simulink model "brake_acc_nodiv"  (Simulink 8.6)
settings: Solver=FixedStepDiscrete  StartTime=0.0  StopTime=30  FixedStep=T_sim  RelTol=1e-6
PostLoadFcn:
  | parameters
undefined symbols (not defined in the file): v0, w0
libraries: simulink x10, lib_abs_nodiv x4, lib_wheel_nodiv x4, lib_brake_torque_cal_nodiv x1, lib_global_brake_ctrl_nodiv x1, lib_spd_estimator_nodiv x1, lib_vehicle_nodiv x1
settings Model: Creator=yt59680  LastModifiedBy=pfj01
settings SolverCC: AutoInsertRateTranBlk=on
settings DebuggingCC: InvalidFcnCallConnMsg=warning  FcnCallInpInsideContextMsg=UseLocalSettings  StrictBusMsg=Warning
settings HardwareCC: TargetBitPerPointer=64  TargetLongLongMode=on  TargetIntDivRoundTo=Zero  TargetEndianess=LittleEndian  TargetWordSize=64  TargetHWDeviceType=MATLAB Host  ProdEqTarget=off
settings RTWCC: SystemTargetFile=rsim.tlc  TemplateMakefile=rsim_default_tmf  Description=Rapid Simulation Target
settings TargetCC: ParMdlRefBuildCompliant=on  ConcurrentExecutionCompliant=on  MatFileLogging=on
settings CustomProperty: DataType=string  Value=Auto

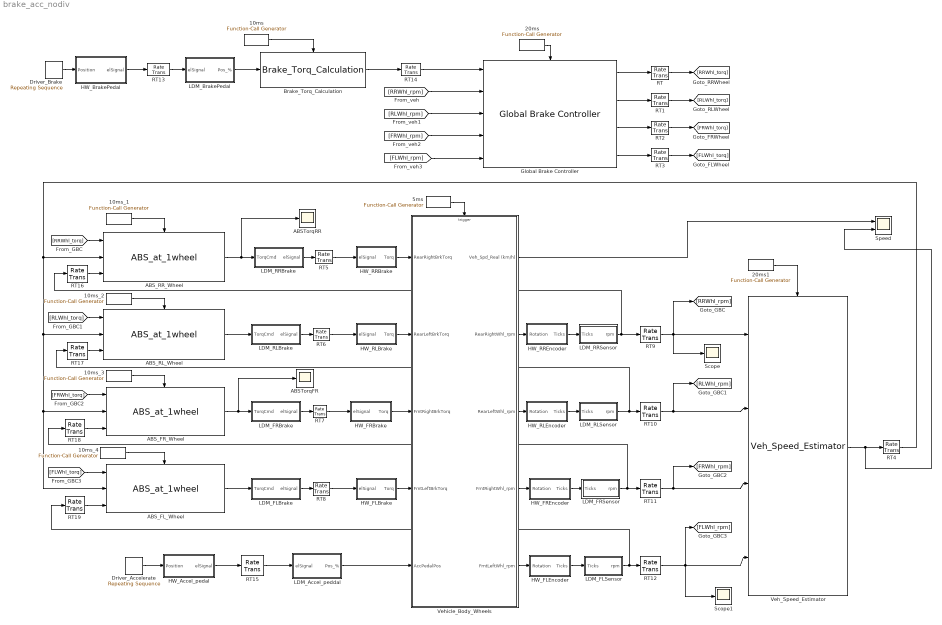
== system brake_acc_nodiv ==
  10ms : simulink/Ports & Subsystems/Function-Call Generator  sample_time=T_brake_pedal  numberOfIterations=1
  10ms_{1..4} (4 alike) : simulink/Ports & Subsystems/Function-Call Generator  sample_time=T_abs  numberOfIterations=1
  20ms : simulink/Ports & Subsystems/Function-Call Generator  sample_time=T_brake_ctrl  numberOfIterations=1
  20ms1 : simulink/Ports & Subsystems/Function-Call Generator  sample_time=T_spd_est  numberOfIterations=1
  5ms : simulink/Ports & Subsystems/Function-Call Generator  sample_time=T_veh  numberOfIterations=1
  ABSTorqFR : Scope
  ABSTorqRR : Scope
  ABS_FL_Wheel : lib_abs_nodiv/ABS_at_1wheel
  ABS_FR_Wheel : lib_abs_nodiv/ABS_at_1wheel
  ABS_RL_Wheel : lib_abs_nodiv/ABS_at_1wheel
  ABS_RR_Wheel : lib_abs_nodiv/ABS_at_1wheel
  Brake_Torq_Calculation : lib_brake_torque_cal_nodiv/Brake_Torq_Calculation
  Driver_Accelerate : simulink/Sources/Repeating Sequence  rep_seq_t=[0 1 10.5 11 100]  rep_seq_y=[0 100 100 0 0]
  Driver_Brake : simulink/Sources/Repeating Sequence  rep_seq_t=[0 19.5 20 100]  rep_seq_y=[0 0 100 100]
  Global Brake Controller : lib_global_brake_ctrl_nodiv/Global Brake Controller
  HW_Accel_pedal : Subsystem
  HW_BrakePedal : Subsystem
  HW_FLBrake : Subsystem
  HW_FLEncoder : Subsystem
  HW_FRBrake : Subsystem
  HW_FREncoder : Subsystem
  HW_RLBrake : Subsystem
  HW_RLEncoder : Subsystem
  HW_RRBrake : Subsystem
  HW_RREncoder : Subsystem
  LDM_Accel_peddal : Subsystem
  LDM_BrakePedal : Subsystem
  LDM_FLBrake : Subsystem
  LDM_FLSensor : Subsystem
  LDM_FRBrake : Subsystem
  LDM_FRSensor : Subsystem
  LDM_RLBrake : Subsystem
  LDM_RLSensor : Subsystem
  LDM_RRBrake : Subsystem
  LDM_RRSensor : Subsystem
  RT{,1..3,5..8,13..15} (11 alike) : RateTransition
  RT{9..12,16..19} (8 alike) : RateTransition  X0=w0*30/pi
  RT4 : RateTransition  X0=v0*3.6
  Scope : Scope
  Scope1 : Scope
  Speed : Scope  NumInputPorts=2
  Veh_Speed_Estimator : lib_spd_estimator_nodiv/Veh_Speed_Estimator
  Vehicle_Body_Wheels : Subsystem
  wires:
  10ms/1 -> Brake_Torq_Calculation/Trigger
  20ms/1 -> Global Brake Controller/Trigger
  Global Brake Controller/1 -> RT/1
  Global Brake Controller/2 -> RT1/1
  Global Brake Controller/3 -> RT2/1
  10ms_1/1 -> ABS_RR_Wheel/Trigger
  ABS_RR_Wheel/1 -> ABSTorqRR/1, LDM_RRBrake/1(TorqCmd)
  RT5/1 -> HW_RRBrake/1(elSignal)
  Vehicle_Body_Wheels/2(RearRightWhl_rpm) -> HW_RREncoder/1(Rotation)
  Global Brake Controller/4 -> RT3/1
  [RRWhl_torq] -> ABS_RR_Wheel/1
  ABS_RL_Wheel/1 -> LDM_RLBrake/1(TorqCmd)
  RT6/1 -> HW_RLBrake/1(elSignal)
  Vehicle_Body_Wheels/3(RearLeftWhl_rpm) -> HW_RLEncoder/1(Rotation)
  [RLWhl_torq] -> ABS_RL_Wheel/1
  ABS_FR_Wheel/1 -> ABSTorqFR/1, LDM_FRBrake/1(TorqCmd)
  RT7/1 -> HW_FRBrake/1(elSignal)
  Vehicle_Body_Wheels/4(FrntRightWhl_rpm) -> HW_FREncoder/1(Rotation)
  [FRWhl_torq] -> ABS_FR_Wheel/1
  ABS_FL_Wheel/1 -> LDM_FLBrake/1(TorqCmd)
  RT8/1 -> HW_FLBrake/1(elSignal)
  Vehicle_Body_Wheels/5(FrntLeftWhl_rpm) -> HW_FLEncoder/1(Rotation)
  [FLWhl_torq] -> ABS_FL_Wheel/1
  Driver_Brake/1 -> HW_BrakePedal/1(Position)
  Brake_Torq_Calculation/1 -> RT14/1
  RT14/1 -> Global Brake Controller/1
  [RRWhl_rpm] -> Global Brake Controller/2
  [RLWhl_rpm] -> Global Brake Controller/3
  [FRWhl_rpm] -> Global Brake Controller/4
  [FLWhl_rpm] -> Global Brake Controller/5
  RT/1 -> [RRWhl_torq]
  RT1/1 -> [RLWhl_torq]
  RT2/1 -> [FRWhl_torq]
  RT3/1 -> [FLWhl_torq]
  RT4/1 -> ABS_FR_Wheel/2, ABS_FL_Wheel/2, ABS_RL_Wheel/2, ABS_RR_Wheel/2
  LDM_RRBrake/1(elSignal) -> RT5/1
  HW_RRBrake/1(Torq) -> Vehicle_Body_Wheels/1(RearRightBrkTorq)
  LDM_RLBrake/1(elSignal) -> RT6/1
  HW_RLBrake/1(Torq) -> Vehicle_Body_Wheels/2(RearLeftBrkTorq)
  LDM_FRBrake/1(elSignal) -> RT7/1
  HW_FRBrake/1(Torq) -> Vehicle_Body_Wheels/3(FrntRightBrkTorq)
  LDM_FLBrake/1(elSignal) -> RT8/1
  HW_FLBrake/1(Torq) -> Vehicle_Body_Wheels/4(FrntLeftBrkTorq)
  HW_RREncoder/1(Ticks) -> LDM_RRSensor/1(Ticks)
  HW_RLEncoder/1(Ticks) -> LDM_RLSensor/1(Ticks)
  HW_FREncoder/1(Ticks) -> LDM_FRSensor/1(Ticks)
  LDM_RRSensor/1(rpm) -> RT16/1, RT9/1
  LDM_RLSensor/1(rpm) -> RT10/1, RT17/1
  LDM_FRSensor/1(rpm) -> RT11/1, RT18/1
  HW_BrakePedal/1(elSignal) -> RT13/1
  LDM_BrakePedal/1(Pos_%) -> Brake_Torq_Calculation/1
  Driver_Accelerate/1 -> HW_Accel_pedal/1(Position)
  5ms/1 -> Vehicle_Body_Wheels/Trigger
  10ms_2/1 -> ABS_RL_Wheel/Trigger
  10ms_3/1 -> ABS_FR_Wheel/Trigger
  10ms_4/1 -> ABS_FL_Wheel/Trigger
  20ms1/1 -> Veh_Speed_Estimator/Trigger
  Veh_Speed_Estimator/1 -> RT4/1, Speed/2
  Vehicle_Body_Wheels/1(Veh_Spd_Real (km/h)) -> Speed/1
  RT13/1 -> LDM_BrakePedal/1(elSignal)
  HW_Accel_pedal/1(elSignal) -> RT15/1
  LDM_Accel_peddal/1(Pos_%) -> Vehicle_Body_Wheels/5(AccPedalPos)
  RT15/1 -> LDM_Accel_peddal/1(elSignal)
  LDM_FLSensor/1(rpm) -> RT19/1, RT12/1
  RT16/1 -> ABS_RR_Wheel/3
  RT17/1 -> ABS_RL_Wheel/3
  RT18/1 -> ABS_FR_Wheel/3
  RT19/1 -> ABS_FL_Wheel/3
  RT9/1 -> Veh_Speed_Estimator/1, [RRWhl_rpm], Scope/1
  RT10/1 -> Veh_Speed_Estimator/2, [RLWhl_rpm]
  RT11/1 -> Veh_Speed_Estimator/3, [FRWhl_rpm]
  HW_FLEncoder/1(Ticks) -> LDM_FLSensor/1(Ticks)
  RT12/1 -> [FLWhl_rpm], Veh_Speed_Estimator/4, Scope1/1

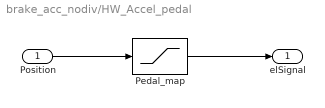
== system brake_acc_nodiv/HW_Accel_pedal ==
  Position : Inport
  Pedal_map : Saturate  UpperLimit=100  LowerLimit=0
  elSignal : Outport
  wires:
  Position/1 -> Pedal_map/1
  Pedal_map/1 -> elSignal/1

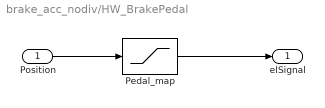
== system brake_acc_nodiv/HW_BrakePedal ==
  Position : Inport
  Pedal_map : Saturate  UpperLimit=100  LowerLimit=0
  elSignal : Outport
  wires:
  Position/1 -> Pedal_map/1
  Pedal_map/1 -> elSignal/1

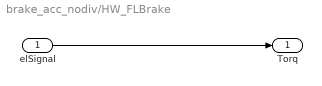
== system brake_acc_nodiv/HW_FLBrake ==
  elSignal : Inport
  Torq : Outport
  wires:
  elSignal/1 -> Torq/1

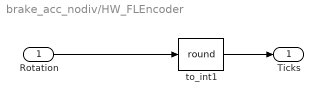
== system brake_acc_nodiv/HW_FLEncoder ==
  Rotation : Inport
  to_int1 : Rounding  Operator=round
  Ticks : Outport
  wires:
  Rotation/1 -> to_int1/1
  to_int1/1 -> Ticks/1

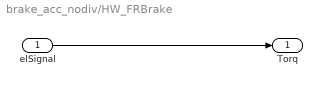
== system brake_acc_nodiv/HW_FRBrake ==
  elSignal : Inport
  Torq : Outport
  wires:
  elSignal/1 -> Torq/1

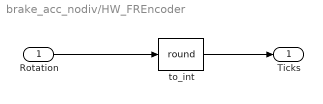
== system brake_acc_nodiv/HW_FREncoder ==
  Rotation : Inport
  to_int : Rounding  Operator=round
  Ticks : Outport
  wires:
  Rotation/1 -> to_int/1
  to_int/1 -> Ticks/1

== system brake_acc_nodiv/HW_RLBrake ==
  elSignal : Inport
  Torq : Outport
  wires:
  elSignal/1 -> Torq/1

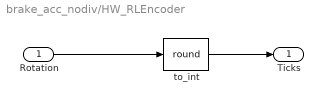
== system brake_acc_nodiv/HW_RLEncoder ==
  Rotation : Inport
  to_int : Rounding  Operator=round
  Ticks : Outport
  wires:
  Rotation/1 -> to_int/1
  to_int/1 -> Ticks/1

== system brake_acc_nodiv/HW_RRBrake ==
  elSignal : Inport
  Torq : Outport
  wires:
  elSignal/1 -> Torq/1

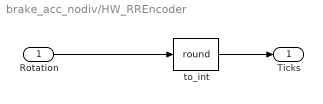
== system brake_acc_nodiv/HW_RREncoder ==
  Rotation : Inport
  to_int : Rounding  Operator=round
  Ticks : Outport
  wires:
  Rotation/1 -> to_int/1
  to_int/1 -> Ticks/1

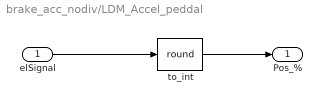
== system brake_acc_nodiv/LDM_Accel_peddal ==
  elSignal : Inport
  to_int : Rounding  Operator=round
  Pos_% : Outport
  wires:
  elSignal/1 -> to_int/1
  to_int/1 -> Pos_%/1

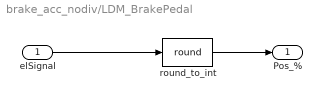
== system brake_acc_nodiv/LDM_BrakePedal ==
  elSignal : Inport
  round_to_int : Rounding  Operator=round
  Pos_% : Outport
  wires:
  elSignal/1 -> round_to_int/1
  round_to_int/1 -> Pos_%/1

== system brake_acc_nodiv/LDM_FLBrake ==
  TorqCmd : Inport
  elSignal : Outport
  wires:
  TorqCmd/1 -> elSignal/1

== system brake_acc_nodiv/LDM_FLSensor ==
  Ticks : Inport
  rpm : Outport
  wires:
  Ticks/1 -> rpm/1

== system brake_acc_nodiv/LDM_FRBrake ==
  TorqCmd : Inport
  elSignal : Outport
  wires:
  TorqCmd/1 -> elSignal/1

== system brake_acc_nodiv/LDM_FRSensor ==
  Ticks : Inport
  rpm : Outport
  wires:
  Ticks/1 -> rpm/1

== system brake_acc_nodiv/LDM_RLBrake ==
  TorqCmd : Inport
  elSignal : Outport
  wires:
  TorqCmd/1 -> elSignal/1

== system brake_acc_nodiv/LDM_RLSensor ==
  Ticks : Inport
  rpm : Outport
  wires:
  Ticks/1 -> rpm/1

== system brake_acc_nodiv/LDM_RRBrake ==
  TorqCmd : Inport
  elSignal : Outport
  wires:
  TorqCmd/1 -> elSignal/1

== system brake_acc_nodiv/LDM_RRSensor ==
  Ticks : Inport
  rpm : Outport
  wires:
  Ticks/1 -> rpm/1

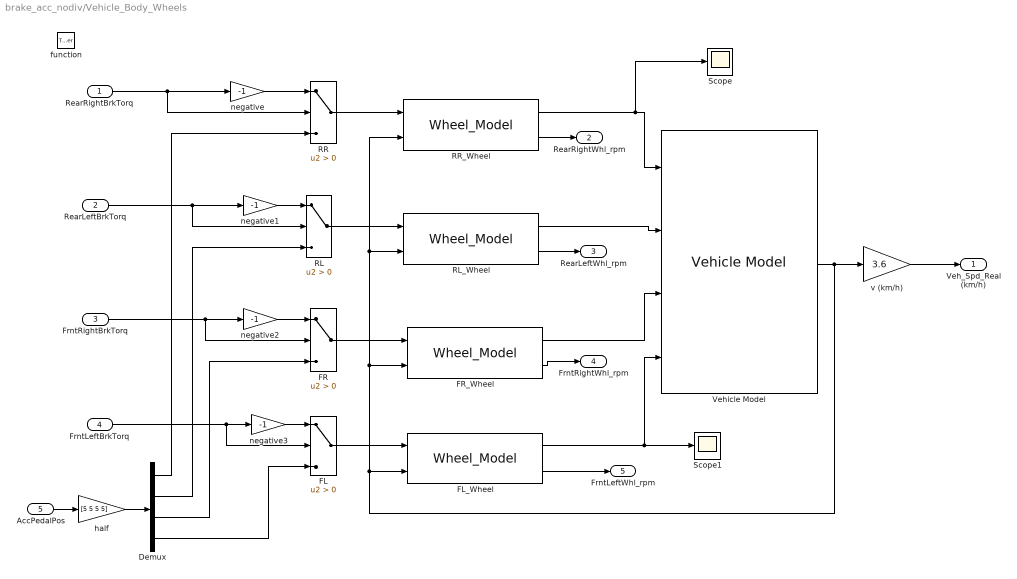
== system brake_acc_nodiv/Vehicle_Body_Wheels ==
  RearRightBrkTorq : Inport
  RearLeftBrkTorq : Inport  Port=2
  FrntRightBrkTorq : Inport  Port=3
  FrntLeftBrkTorq : Inport  Port=4
  AccPedalPos : Inport  Port=5
  function : TriggerPort  TriggerType=function-call  VariantControl=Variant
  Demux : Demux
  FL : Switch  Criteria=u2 > Threshold
  FL_Wheel : lib_wheel_nodiv/Wheel_Model
      link override friction_force_N: OutMax=1000000
  FR : Switch  Criteria=u2 > Threshold
  FR_Wheel : lib_wheel_nodiv/Wheel_Model
      link override friction_force_N: OutMax=1000000
  RL : Switch  Criteria=u2 > Threshold
  RL_Wheel : lib_wheel_nodiv/Wheel_Model
      link override friction_force_N: OutMax=1000000
  RR : Switch  Criteria=u2 > Threshold
  RR_Wheel : lib_wheel_nodiv/Wheel_Model
      link override friction_force_N: OutMax=100000
  Scope : Scope
  Scope1 : Scope
  Vehicle Model : lib_vehicle_nodiv/Vehicle Model
  half : Gain  Gain=[5 5 5 5]  ParamDataTypeStr=double
  negative{,1..3} (4 alike) : Gain  Gain=-1
  v (km/h) : Gain  Gain=3.6  OutMin=0  OutMax=200
  Veh_Spd_Real (km/h) : Outport
  RearRightWhl_rpm : Outport  Port=2
  RearLeftWhl_rpm : Outport  Port=3
  FrntRightWhl_rpm : Outport  Port=4
  FrntLeftWhl_rpm : Outport  Port=5
  wires:
  Vehicle Model/1 -> v (km/h)/1, RR_Wheel/2, RL_Wheel/2, FR_Wheel/2, FL_Wheel/2
  RR_Wheel/2 -> RearRightWhl_rpm/1
  RR_Wheel/1 -> Scope/1, Vehicle Model/1
  RL_Wheel/2 -> RearLeftWhl_rpm/1
  RL_Wheel/1 -> Vehicle Model/2
  FR_Wheel/2 -> FrntRightWhl_rpm/1
  FR_Wheel/1 -> Vehicle Model/3
  FL_Wheel/1 -> Scope1/1, Vehicle Model/4
  AccPedalPos/1 -> half/1
  FR/1 -> FR_Wheel/1
  FrntRightBrkTorq/1 -> FR/2, negative2/1
  FL/1 -> FL_Wheel/1
  FrntLeftBrkTorq/1 -> FL/2, negative3/1
  RR/1 -> RR_Wheel/1
  RearRightBrkTorq/1 -> RR/2, negative/1
  RL/1 -> RL_Wheel/1
  RearLeftBrkTorq/1 -> RL/2, negative1/1
  half/1 -> Demux/1
  Demux/1 -> RR/3
  Demux/2 -> RL/3
  Demux/3 -> FR/3
  Demux/4 -> FL/3
  v (km/h)/1 -> Veh_Spd_Real (km/h)/1
  negative/1 -> RR/1
  negative1/1 -> RL/1
  negative2/1 -> FR/1
  negative3/1 -> FL/1
  FL_Wheel/2 -> FrntLeftWhl_rpm/1
